simulink model "mbed_nucleo_f303_i2c_peripherals"  (R2015a)
settings: Solver=FixedStepDiscrete  SolverMode=SingleTasking  StartTime=0.0  StopTime=10.0  FixedStep=.1  RelTol=1e-3
undefined symbols (not defined in the file or in its folder): x1
libraries: mbed_lib x13, simulink x2, mbed_targets_stm_disco_f407 x2, mbed_targets_stm_nucleo_f446 x1
settings Model: Creator=Stuv  LastModifiedBy=Stuv
settings OptimizationCC: OptimizeModelRefInitCode=on  LifeSpan=1
settings HardwareCC: ProdLargestAtomicInteger=Long  ProdLargestAtomicFloat=Double  ProdEndianess=LittleEndian  ProdHWDeviceType=ARM Compatible->ARM Cortex
settings RTWCC: SystemTargetFile=mbed.tlc  TemplateMakefile=mbed.tmf  Description=Mbed Target (Embedded Target)  TargetLang=C++
settings CodeAppCC: IgnoreCustomStorageClasses=off
settings STFCustomTargetCC: CombineOutputUpdateFcns=on  SupportContinuousTime=off  SupportVariableSizeSignals=off  SystemTargetFile=mbed.tlc
settings ERTTargetCC: SupportContinuousTime=off  SupportVariableSizeSignals=off  ERTCustomFileTemplate=mbed_file_process.tlc

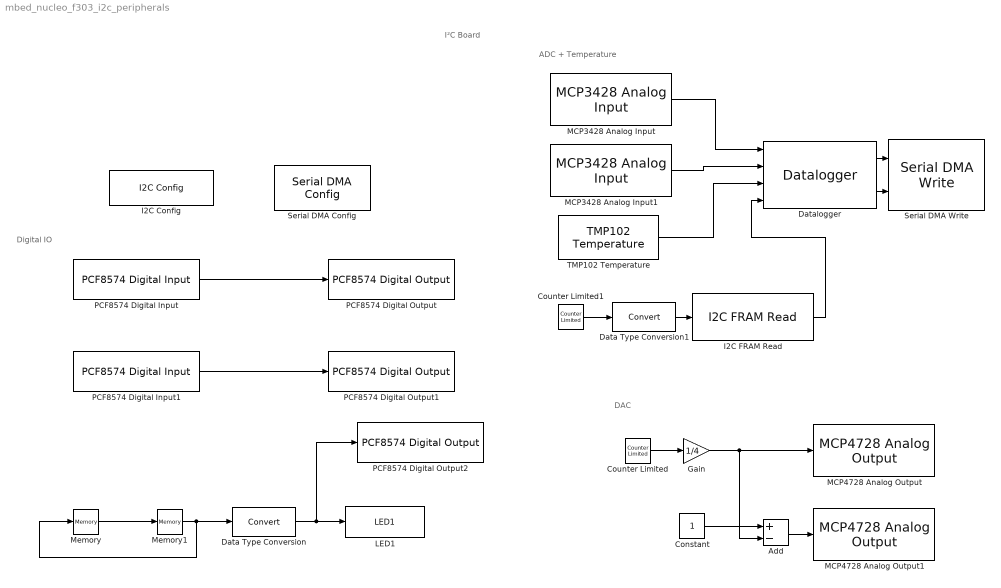
== system mbed_nucleo_f303_i2c_peripherals ==
  note: I²C Board
  note: Digital IO
  note: ADC + Temperature
  note: DAC
  Add : Sum  Inputs=+-
  Constant : Constant  OutDataTypeStr=single
  Counter Limited : simulink/Sources/Counter Limited  uplimit=4  tsamp=-1
  Counter Limited1 : simulink/Sources/Counter Limited  uplimit=11  tsamp=-1
  Data Type Conversion : DataTypeConversion
  Data Type Conversion1 : DataTypeConversion
  Datalogger : mbed_lib/Utilities/Datalogger  TypeInputPorts={ 'single' 1 'single' 1 'single' 1 'uint8' 1 }  TypeOfInputs={'1*single','1*single','1*single','1*uint8'}  BufferSize=40  errEn=off  SampleTime=-1
  Gain : Gain  Gain=1/4  OutDataTypeStr=single
  I2C Config : mbed_lib/I2C/I2C Config  Priority=0  I2cPort=1  SParameter6=100000  SParameter2=B  SParameter3=7  SParameter4=B  SParameter5=6
  I2C FRAM Read : mbed_lib/I2C/I2C FRAM Read  I2cPort=1  EnableError=off
  LED1 : mbed_targets_stm_nucleo_f446/LED1  Parameter1=0
  MCP3428 Analog Input : mbed_lib/I2C/MCP3428 Analog Input  I2cPort=1  SubAddress=0xD0  EnableError=off  Channel=1  Mode=voltage  Resolution=12 bit  Gain=x1
  MCP3428 Analog Input1 : mbed_lib/I2C/MCP3428 Analog Input  I2cPort=1  SubAddress=0xD2  EnableError=off  Channel=1  Mode=voltage  Resolution=12 bit  Gain=x1
  MCP4728 Analog Output : mbed_lib/I2C/MCP4728 Analog Output  I2cPort=1  SubAddress=0xC0  EnableError=off  Channel=A  Mode=relative  RefVoltage=External  Gain=x1
  MCP4728 Analog Output1 : mbed_lib/I2C/MCP4728 Analog Output  I2cPort=1  SubAddress=0xC0  EnableError=off  Channel=B  Mode=relative  RefVoltage=External  Gain=x1
  Memory : Memory  X0=1  InheritSampleTime=on
  Memory1 : Memory  InheritSampleTime=on
  PCF8574 Digital Input : mbed_lib/I2C/PCF8574 Digital Input  I2cPort=1  SubAddress=0x40  PinNumber=Pin 6  EnableError=off
  PCF8574 Digital Input1 : mbed_lib/I2C/PCF8574 Digital Input  I2cPort=1  SubAddress=0x72  PinNumber=Pin 7  EnableError=off
  PCF8574 Digital Output : mbed_lib/I2C/PCF8574 Digital Output  I2cPort=1  SubAddress=0x40  PinNumber=Pin 0  EnableError=off
  PCF8574 Digital Output1 : mbed_lib/I2C/PCF8574 Digital Output  I2cPort=1  SubAddress=0x40  PinNumber=Pin 1  EnableError=off
  PCF8574 Digital Output2 : mbed_lib/I2C/PCF8574 Digital Output  I2cPort=1  SubAddress=0x40  PinNumber=Pin 2  EnableError=off
  Serial DMA Config : mbed_targets_stm_disco_f407/Serial DMA Config  SerialPort=2  TxPort=A  TxPin=2  RxPort=A  RxPin=3  BaudRate=115200
  Serial DMA Write : mbed_targets_stm_disco_f407/Serial DMA Write  SerialPort=2  numData=on  SampleTime=-1
  TMP102 Temperature : mbed_lib/I2C/TMP102 Temperature  I2cPort=1  SubAddress=0x90  SampleRate=4 Hz  EnableError=off
  wires:
  Datalogger/1 -> Serial DMA Write/1
  Datalogger/2 -> Serial DMA Write/2
  MCP3428 Analog Input1/1 -> Datalogger/2
  Memory/1 -> Memory1/1
  Memory1/1 -> Data Type Conversion/1, Memory/1
  Data Type Conversion/1 -> PCF8574 Digital Output2/1, LED1/1
  TMP102 Temperature/1 -> Datalogger/3
  PCF8574 Digital Input1/1 -> PCF8574 Digital Output1/1
  PCF8574 Digital Input/1 -> PCF8574 Digital Output/1
  Counter Limited/1 -> Gain/1
  Gain/1 -> MCP4728 Analog Output/1, Add/2
  Add/1 -> MCP4728 Analog Output1/1
  Constant/1 -> Add/1
  MCP3428 Analog Input/1 -> Datalogger/1
  Counter Limited1/1 -> Data Type Conversion1/1
  Data Type Conversion1/1 -> I2C FRAM Read/1
  I2C FRAM Read/1 -> Datalogger/4
